simulink subsystem "Gas_prop_valve_R2024a"  (R2024a)
settings: Solver=VariableStepAuto  StartTime=0.0  StopTime=10.0  RelTol=1e-3
undefined symbols (not defined in the file or in its folder): Gas_prop_valve_gain, Gas_prop_valve_rate_speed
libraries: SimscapeFluids_lib x2, nesl_utility x2
settings Model: Creator=MW  LastModifiedBy=MW

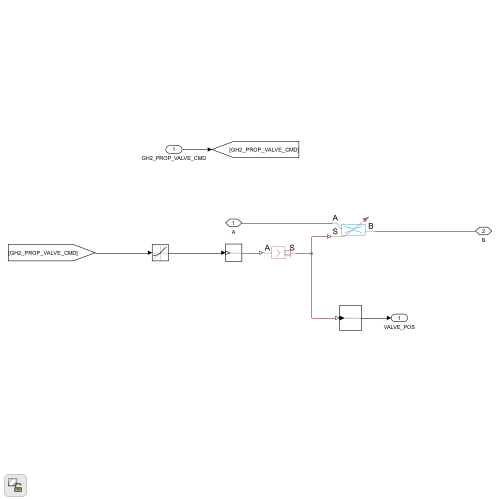
[thumbnail: Simulink's stored preview of the top-level diagram]
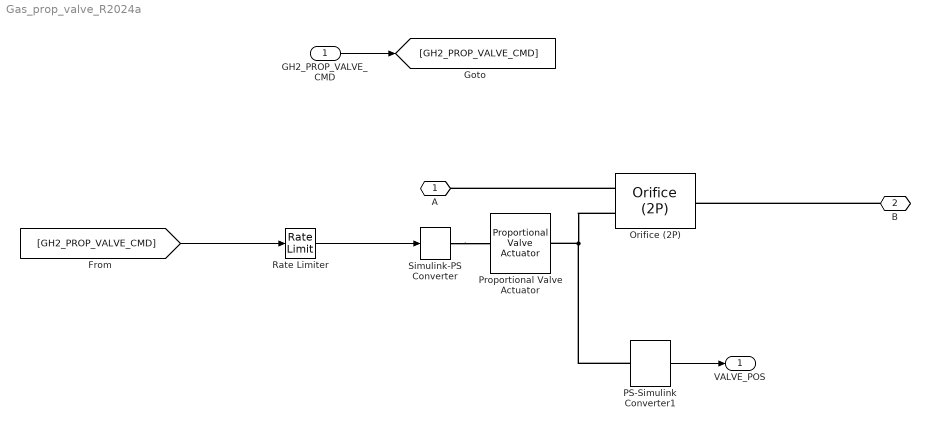
== system Gas_prop_valve_R2024a ==
  GH2_PROP_VALVE_CMD : Inport
  Orifice (2P) : SimscapeFluids_lib/Two-Phase Fluid/Valves & Orifices/Orifice (2P)  orifice_type=foundation.enum.constant_variable.variable  constant_liquid_orifice_parameterization=fluids.two_phase_fluid.valves_orifices.enum.LiquidConstantOrificeParameterization.Area  variable_liquid_orifice_parameterization=fluids.two_phase_fluid.valves_orifices.enum.LiquidOrificeParameterization.LinearArea  mdot_nominal_constant=0.1 kg/s  delta_p_nominal_constant=0.001 MPa  orifice_area_constant=1e-4 m^2  S_min=0 m  del_S=Gas_prop_valve_stroke m  open_orientation=fluids.two_phase_fluid.valves_orifices.enum.OrificeOrientation.Positive  mdot_nominal_max=0.1 kg/s  delta_p_nominal_max=0.001 MPa  orifice_area_max=Gas_prop_valve_orifice_area m^2  S_TLU=[0, .002, .004, .007, .017] m  orifice_area_TLU=[1e-10, 2e-05, 4e-05, 6e-05, 8e-05, .0001] m^2  energy_spec=foundation.enum.energy_spec.temperature  p_inlet=0.101325 MPa  T_inlet=293.15 K  x_inlet=0  alpha_inlet=0  h_inlet=400 kJ/kg  u_inlet=400 kJ/kg  Cd=Gas_prop_valve_discharge_coeff  pressure_recovery=false  leakage_fraction=Gas_prop_valve_leakage  smoothing_factor=0.01  B_lam=Gas_prop_valve_laminar_p_ratio  tau_x=0.1 s  area=supply_pipe_inner_area m^2  vapor_orifice_parameterization=fluids.two_phase_fluid.valves_orifices.enum.VaporOrificeParameterization.Cv  opening_characteristic=fluids.two_phase_fluid.valves_orifices.enum.OpeningCharacteristics.Linear  Cv_constant=4  Cv_max=4  S_Cv_TLU=[0, .003, .006, .009, .012, .015] m  Cv_TLU=[1e-06, .8, 1.6, 2.4, 3.2, 4]  xT_Cv=0.7  Kv_constant=3.6  Kv_max=3.6  S_Kv_TLU=[0, .003, .006, .009, .012, .015] m  Kv_TLU=[1e-06, .72, 1.44, 2.16, 2.88, 3.6]  xT_Kv=0.7  S_orifice_area_TLU=[0, .003, .006, .009, .012, .015] m
      settings: InternalSimscapePortConfiguration="{\"Bottom\":[],\"Left\":[{\"id\":\"A\",\"label\":\"A\",\"type\":\"foundation.two_phase_fluid.two_phase_fluid\"},{\"id\":\"S\",\"label\":\"S\",\"type\":\"input\"}],\"Right\":[{\"id\":\"B\",\"label\":\"B\",\"type\":\"foundation.two_phase_fluid.two_phase_fluid\"}],\"Top\":[]}"
  PS-Simulink Converter1 : nesl_utility/PS-Simulink Converter  PhysicalDomain=network_engine_domain  SubClassName=ps_output  LeftPortType=input  RightPortType=output  PseudoPeriodic=off  Frequencies=[]  VectorFormat=inherit  Unit=inherit  AffineConversion=off
  Proportional Valve Actuator : SimscapeFluids_lib/Valve Actuators/Proportional Valve Actuator  gain=Gas_prop_valve_gain m  time_constant=0.01 s  valve_stroke=Gas_prop_valve_stroke m
      settings: InternalSimscapePortConfiguration="{\"Bottom\":[],\"Left\":[{\"id\":\"A\",\"label\":\"A\",\"type\":\"input\"}],\"Right\":[{\"id\":\"S\",\"label\":\"S\",\"type\":\"output\"}],\"Top\":[]}"
  Rate Limiter : RateLimiter  RisingSlewLimit=Gas_prop_valve_rate_speed  FallingSlewLimit=-Gas_prop_valve_rate_speed  SampleTimeMode=inherited
  Simulink-PS Converter : nesl_utility/Simulink-PS Converter  PhysicalDomain=network_engine_domain  SubClassName=ps_input  LeftPortType=input  RightPortType=output  PseudoPeriodic=off  Frequencies=[]  NoiseDistribution=none  NoiseParameters=[]  Unit=1  AffineConversion=off  FilteringAndDerivatives=provide  SimscapeFilterOrder=1  InputFilterTimeConstant=0.001  UdotUserProvided=0
  A : PMIOPort  Side=Left
  B : PMIOPort  Port=2  Side=Left
  VALVE_POS : Outport
  wires:
  GH2_PROP_VALVE_CMD/1 -> [GH2_PROP_VALVE_CMD]
  PS-Simulink Converter1/1 -> VALVE_POS/1
  [GH2_PROP_VALVE_CMD] -> Rate Limiter/1
  Rate Limiter/1 -> Simulink-PS Converter/1
  connections:
  PS-Simulink Converter1/LConn1 -- Orifice (2P)/LConn2 -- Proportional Valve Actuator/RConn1
  B/RConn1 -- Orifice (2P)/RConn1
  Orifice (2P)/LConn1 -- A/RConn1
  Simulink-PS Converter/RConn1 -- Proportional Valve Actuator/LConn1
